simulink model "RealimentacaoPadrao"  (R2019a)
settings: Solver=VariableStepAuto  StartTime=0.0  StopTime=10  RelTol=1e-3
undefined symbols (not defined in the file): A, B, C, K
settings Model: Creator=Cliente  LastModifiedBy=Cliente

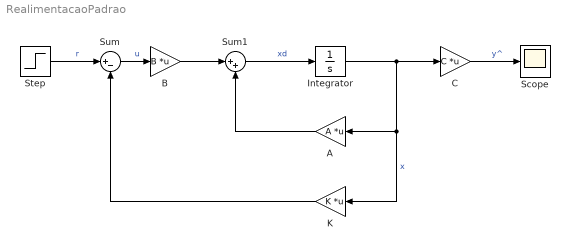
== system RealimentacaoPadrao ==
  A : Gain  Gain=A  Multiplication=Matrix(K*u) (u vector)
  B : Gain  Gain=B  Multiplication=Matrix(K*u)
  C : Gain  Gain=C  Multiplication=Matrix(K*u) (u vector)
  Integrator : Integrator
  K : Gain  Gain=K  Multiplication=Matrix(K*u) (u vector)
  Scope : Scope
  Step : Step  Time=0  SampleTime=0
  Sum : Sum  Inputs=|+-
  Sum1 : Sum  Inputs=|++
  wires:
  Integrator/1 -> K/1, A/1, C/1  "x"
  Sum1/1 -> Integrator/1  "xd"
  B/1 -> Sum1/1
  Sum/1 -> B/1  "u"
  Step/1 -> Sum/1  "r"
  A/1 -> Sum1/2
  K/1 -> Sum/2
  C/1 -> Scope/1  "y^"
